simulink model "comppresser"  (Simulink 7.9)
settings: Solver=ode45  StartTime=0.0  StopTime=2  RelTol=1e-3
libraries: dspsrcs4 x1, simulink x1
settings Model: Creator=ArunKB  LastModifiedBy=ArunKB

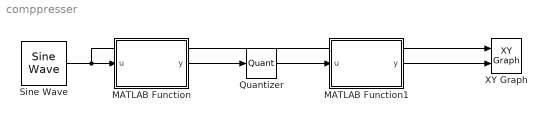
== system comppresser ==
  MATLAB Function : MATLAB Function  TreatAsAtomicUnit=on
  MATLAB Function1 : MATLAB Function  TreatAsAtomicUnit=on
  Quantizer : Quantizer
  Sine Wave : dspsrcs4/Sine Wave  Amplitude=10  Frequency=1  Phase=0  SampleMode=Discrete  OutComplex=Real  CompMethod=Trigonometric fcn  TableSize=Speed  SampleTime=1/1000  SamplesPerFrame=1  ResetState=Restart at time zero  dataType=double  wordLen=16  udDataType=sfix(16)  fracBitsMode=Best precision  numFracBits=15  OutDataTypeStr=double  LastOutDataTypeStr=double
  XY Graph : simulink/Sinks/XY Graph  xmin=-3  xmax=3  ymin=-10  ymax=10  st=-1
  wires:
  Sine Wave/1 -> MATLAB Function/1(u), XY Graph/1
  MATLAB Function/1(y) -> Quantizer/1
  Quantizer/1 -> MATLAB Function1/1(u)
  MATLAB Function1/1(y) -> XY Graph/2

== matlab function MATLAB Function1 ==
  data: u input double; y output double
function y = fcn(u)
%#codegen
c=0;
if(abs(u)<2)
    c=u/2;
elseif(u>2)
    c=3*u/2-2;
elseif(u<-2)
    c=3*u/2+2;
end
y=c;
end

== matlab function MATLAB Function ==
  data: u input double; y output double
function y = fcn(u)
%#codegen
c=0;
if(abs(u)<1)
    c=2*u;
elseif(u>1)
    c=2*u/3+4/3;
elseif(u<-1)
    c=2*u/3-4/3;
end
y=c;
end
